simulink model "sim_dgl_Ofen"  (R2021b)
settings: Solver=ode45  StartTime=0.0  StopTime=10.0  RelTol=1e-3  EnableMultiTasking=on
values from neighbouring files (symbols this model uses):
  T_Ofen = 800    [test_simulink.m]    (also in ueb_simulink_ofen.m)
  T_w_0 = 20    [test_simulink.m]    (also in ueb_simulink_ofen.m)
  Tau = La/Ra    (= 0.00267462686567)    [test_DC_Motor.m]    (also in test_simulink.m = 10319.9174407; ueb_simulink_ofen.m = 10319.9174407)
settings Model: Creator=dep02378  LastModifiedBy=Horst
settings SolverCC: AlgebraicLoopSolver=TrustRegion
settings DataIOCC: LimitDataPoints=on  SaveFormat=Array  SignalLoggingSaveFormat=ModelDataLogs  ReturnWorkspaceOutputs=off
settings OptimizationCC: ExpressionDepthLimit=2147483647  LifeSpan=inf
settings DebuggingCC: UnderspecifiedInitializationDetection=Classic  MergeDetectMultiDrivingBlocksExec=none  FcnCallInpInsideContextMsg=warning  StateNameClashWarn=warning  SFUnexpectedBacktrackingDiag=warning  SFNoUnconditionalDefaultTransitionDiag=warning  SFExecutionAtInitializationDiag=none  SFMachineParentedDataDiag=warning  ArithmeticOperatorsInVariantConditions=warning
settings HardwareCC: ProdBitPerPointer=32  ProdBitPerSizeT=32  ProdBitPerPtrDiffT=32  ProdLargestAtomicFloat=None  ProdIntDivRoundTo=Undefined  ProdEndianess=Unspecified  ProdWordSize=32  ProdHWDeviceType=32-bit Generic
settings ModelReferenceCC: PropagateSignalLabelsOutOfModel=off
settings SFSimCC: SimUseLocalCustomCode=off  CustomCodeUndefinedFunction=UseInterfaceOnly
settings RTWCC: RTWUseLocalCustomCode=off
settings CodeAppCC: StateflowObjectComments=on
settings GRTTargetCC: TargetLangStandard=C89/C90 (ANSI)
settings ConfigComp: CovMetricSettings=dw  CovSaveCumulativeToWorkspaceVar=on  CovSaveSingleToWorkspaceVar=on  CovExternalEMLEnable=off

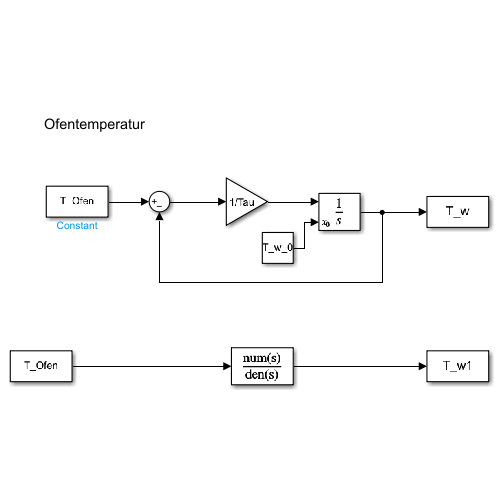
[thumbnail: Simulink's stored preview of the top-level diagram]
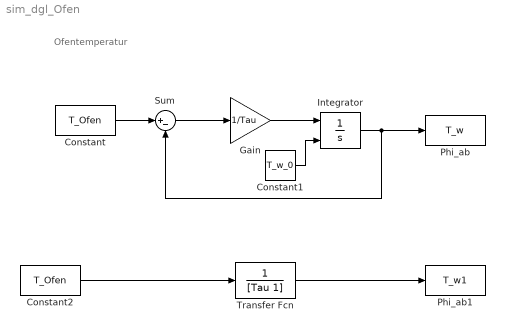
== system sim_dgl_Ofen ==
  note: Ofentemperatur
  Constant : Constant  Value=T_Ofen
  Constant1 : Constant  Value=T_w_0
  Constant2 : Constant  Value=T_Ofen
  Gain : Gain  Gain=1/Tau
  Integrator : Integrator  InitialConditionSource=external
  Phi_ab : ToWorkspace  VariableName=T_w  SampleTime=-1
  Phi_ab1 : ToWorkspace  VariableName=T_w1  SampleTime=-1
  Sum : Sum  Inputs=|+-
  Transfer Fcn : TransferFcn  Denominator=[Tau 1]
  wires:
  Constant/1 -> Sum/1
  Sum/1 -> Gain/1
  Gain/1 -> Integrator/1
  Integrator/1 -> Sum/2, Phi_ab/1
  Constant1/1 -> Integrator/2
  Transfer Fcn/1 -> Phi_ab1/1
  Constant2/1 -> Transfer Fcn/1
